simulink model "Lab_8_2"  (R2023a)
settings: Solver=VariableStepAuto  StartTime=0.0  StopTime=10.0  RelTol=1e-3
libraries: dspfdesign x1, dspsigops x1
settings Model: Creator=mluser  LastModifiedBy=mluser

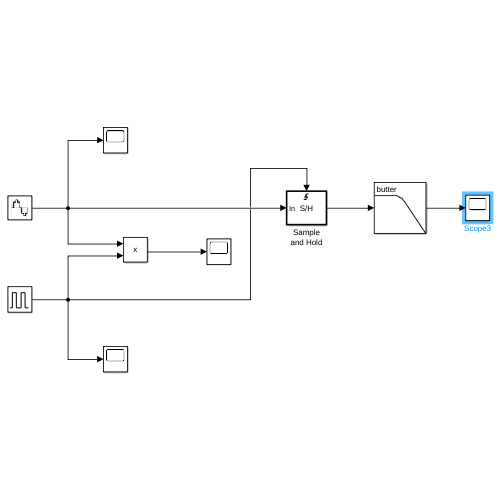
[thumbnail: Simulink's stored preview of the top-level diagram]
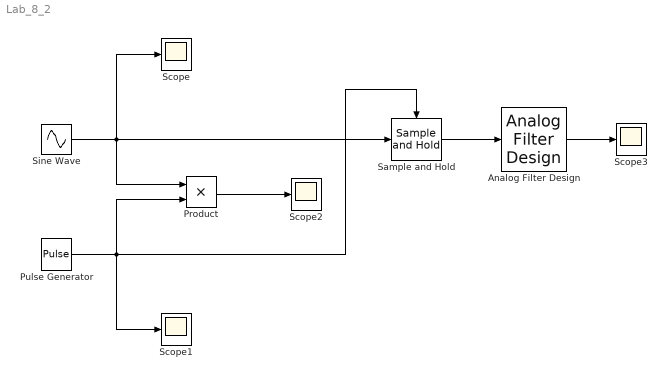
== system Lab_8_2 ==
  Analog Filter Design : dspfdesign/Analog Filter Design  method=Butterworth  filttype=Lowpass  N=3  Wlo=4  Whi=80  Rp=2  Rs=40
  Product : Product
  Pulse Generator : DiscretePulseGenerator  PulseType=Time based  Period=0.8  PulseWidth=50
  Sample and Hold : dspsigops/Sample and Hold  trig=Rising edge  initCond=0  latchinput=off
  Scope{,1..3} (4 alike) : Scope
  Sine Wave : Sin  SampleTime=0.01
  wires:
  Sine Wave/1 -> Product/1, Sample and Hold/1, Scope/1
  Product/1 -> Scope2/1
  Pulse Generator/1 -> Sample and Hold/Trigger, Product/2, Scope1/1
  Sample and Hold/1 -> Analog Filter Design/1
  Analog Filter Design/1 -> Scope3/1
